simulink model "ABS_simulink_model"  (R2023a)
settings: Solver=VariableStepAuto  StartTime=0.0  StopTime=20  RelTol=1e-3
libraries: simulink x2
settings Model: Creator=siddh  LastModifiedBy=siddh
settings ModelReferenceCC: EnableRefExpFcnMdlSchedulingChecks=on

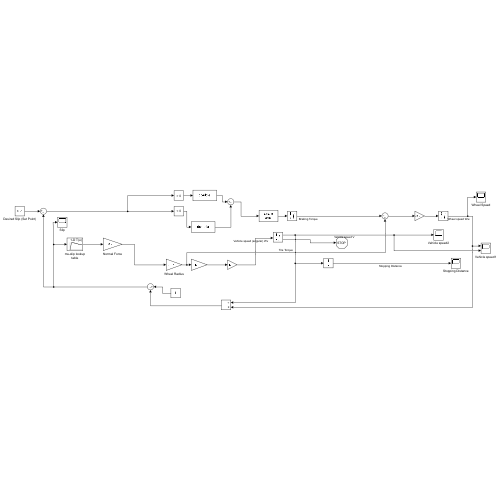
[thumbnail: Simulink's stored preview of the top-level diagram]
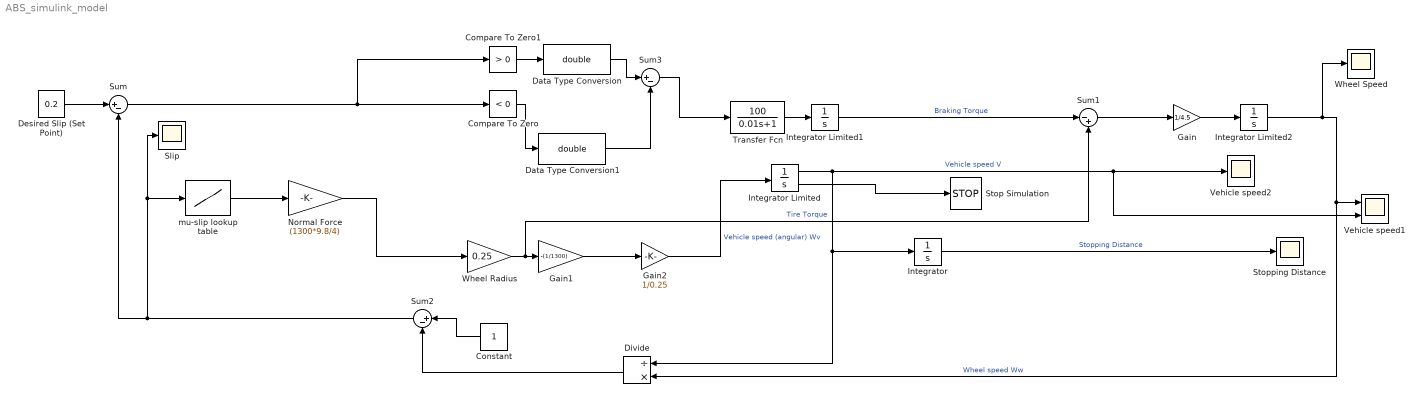
== system ABS_simulink_model ==
  Compare To Zero : simulink/Logic and Bit Operations/Compare To Zero  relop=<  OutDataTypeStr=boolean
  Compare To Zero1 : simulink/Logic and Bit Operations/Compare To Zero  relop=>  OutDataTypeStr=boolean
  Constant : Constant
  Data Type Conversion : DataTypeConversion  OutDataTypeStr=double  SaturateOnIntegerOverflow=off
  Data Type Conversion1 : DataTypeConversion  OutDataTypeStr=double  SaturateOnIntegerOverflow=off
  "Desired Slip (Set Point) " : Constant  Value=0.2
  Divide : Product  Inputs=/*
  Gain : Gain  Gain=1/4.5
  Gain1 : Gain  Gain=-(1/1300)
  Gain2 : Gain  Gain=1/0.25
  Integrator : Integrator
  Integrator Limited : Integrator  InitialCondition=30  LimitOutput=on  UpperSaturationLimit=1000  LowerSaturationLimit=0  ShowSaturationPort=on
  Integrator Limited1 : Integrator  LimitOutput=on  UpperSaturationLimit=1500  LowerSaturationLimit=0
  Integrator Limited2 : Integrator  InitialCondition=30  LimitOutput=on  UpperSaturationLimit=1000  LowerSaturationLimit=0
  Normal Force : Gain  Gain=(1300*9.8/4)
  "Slip " : Scope
  Stop Simulation : Stop
  Stopping Distance : Scope
  Sum : Sum  Inputs=|+-
  Sum1 : Sum  Inputs=|-+
  Sum2 : Sum  Inputs=|+-
  Sum3 : Sum  Inputs=|+-
  Transfer Fcn : TransferFcn  Numerator=[100]  Denominator=[0.01 1]
  Vehicle speed1 : Scope  NumInputPorts=2
  Vehicle speed2 : Scope
  Wheel Radius : Gain  Gain=0.25
  Wheel Speed : Scope
  mu-slip lookup table : Lookup_n-D  NumberOfTableDimensions=1  BreakpointsForDimension1=[0,0.05,0.1,0.15,0.2,0.25,0.3,0.35,0.4,0.45,0.5,0.55,0.60,0.65,0.70,0.75,0.80,0.85,0.90,0.95,1]  Table=[0,0.4,0.8,0.97,1,0.98,0.96,0.94,0.92,0.9,0.88,0.855,0.83,0.81,0.79,0.77,0.75,0.73,0.72,0.71,0.7]  InternalRulePriority=Speed  RndMeth=Simplest
  wires:
  Wheel Radius/1 -> Sum1/2, Gain1/1  "Tire Torque"
  Integrator Limited/1 -> Divide/1, Integrator/1, Vehicle speed2/1, Vehicle speed1/2  "Vehicle speed V"
  "Desired Slip (Set Point) "/1 -> Sum/1
  mu-slip lookup table/1 -> Normal Force/1
  Sum2/1 -> "Slip "/1, mu-slip lookup table/1, Sum/2
  Normal Force/1 -> Wheel Radius/1
  Integrator/1 -> Stopping Distance/1  "Stopping Distance"
  Gain1/1 -> Gain2/1
  Gain2/1 -> Integrator Limited/1  "Vehicle speed (angular) Wv"
  Integrator Limited/2 -> Stop Simulation/1
  Integrator Limited2/1 -> Divide/2, Vehicle speed1/1, Wheel Speed/1  "Wheel speed Ww"
  Gain/1 -> Integrator Limited2/1
  Sum1/1 -> Gain/1
  Constant/1 -> Sum2/1
  Divide/1 -> Sum2/2
  Data Type Conversion1/1 -> Sum3/2
  Data Type Conversion/1 -> Sum3/1
  Compare To Zero1/1 -> Data Type Conversion/1
  Compare To Zero/1 -> Data Type Conversion1/1
  Sum/1 -> Compare To Zero/1, Compare To Zero1/1
  Sum3/1 -> Transfer Fcn/1
  Integrator Limited1/1 -> Sum1/1  "Braking Torque"
  Transfer Fcn/1 -> Integrator Limited1/1
